simulink model "SSNominalModelDirectDigital"  (R2020b)
settings: Solver=ode45  StartTime=0.0  StopTime=10.0  FixedStep=0.0001  MaxStep=0.0001  RelTol=1e-3
values from neighbouring files (symbols this model uses):
  Ts = T2    (= 0.01)    [PIDAntiWindupDigital.m]    (also in PIDDigital.m = 0.001; StateSpaceControllerNominalCont.m = 0.001; StateSpaceControllerNominalDigital.m = 0.001; StateSpaceControllerNominalDirectDigital.m = 0.05)
settings Model: Creator=umberto  LastModifiedBy=umberto
settings SolverCC: AlgebraicLoopSolver=LineSearch

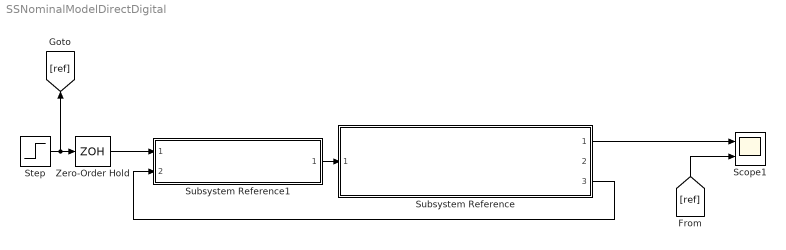
== system SSNominalModelDirectDigital ==
  Scope1 : Scope  NumInputPorts=2
  Step : Step  After=50  SampleTime=0
  Subsystem Reference : Subsystem  ReferencedSubsystem=DCServoMotor_SubSystem
  Subsystem Reference1 : Subsystem  ReferencedSubsystem=RegulatorDirectDigital_SubSystem
  Zero-Order Hold : ZeroOrderHold  SampleTime=Ts
  wires:
  Subsystem Reference/3 -> Subsystem Reference1/2
  [ref] -> Scope1/2
  Subsystem Reference/1 -> Scope1/1
  Step/1 -> Zero-Order Hold/1, [ref]
  Subsystem Reference1/1 -> Subsystem Reference/1
  Zero-Order Hold/1 -> Subsystem Reference1/1
